simulink model "stateflow_ex"  (R2023b)
settings: Solver=VariableStepAuto  StartTime=0.0  StopTime=10.0  RelTol=1e-3
InitFcn:
  | para
undefined symbols (not defined in the file): condition
settings Model: Creator=SJ  LastModifiedBy=SJ

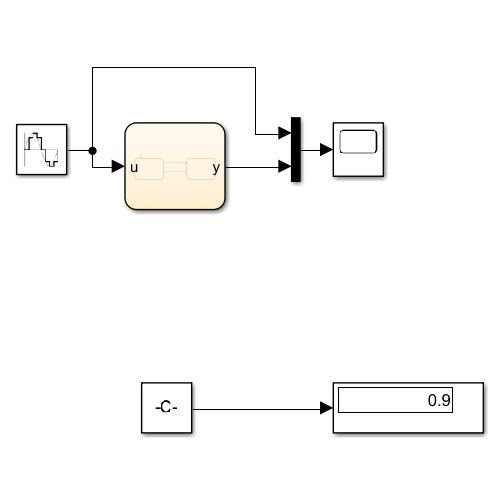
[thumbnail: Simulink's stored preview of the top-level diagram]
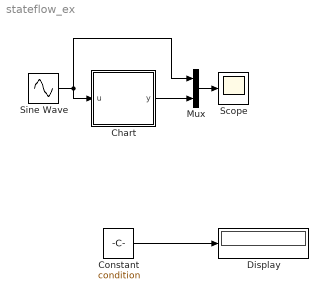
== system stateflow_ex ==
  Chart : Stateflow chart  TreatAsAtomicUnit=on
  Constant : Constant  Value=condition
  Display : Display
  Mux : Mux  Inputs=2
  Scope : Scope
  Sine Wave : Sin  SampleTime=0.1
  wires:
  Sine Wave/1 -> Mux/1, Chart/1(u)
  Mux/1 -> Scope/1
  Chart/1(y) -> Mux/2
  Constant/1 -> Display/1

== stateflow chart stateflow_ex/Chart ==
  state stateA
    en, du:
    y=u;
  state stateB
    en, du:
    y=0;
  (default) -> stateA
  stateA -> stateB : [abs(u)>condition]
  stateB -> stateA : [abs(u)<=condition]
  data: u input; y output; condition parameter double
